simulink model "fixed_point_pi_q14"  (R2023b)
settings: Solver=FixedStepDiscrete  StartTime=0.0  StopTime=0.02  FixedStep=5.0000000000000002e-05  RelTol=1e-3
values from neighbouring files (symbols this model uses):
  feedback_step = 0.2    [build_fixed_point_pi_q14_model.m]
  kidt = Ki * Ts    (= 0.005)    [build_fixed_point_pi_q14_model.m]
  Kp = 10    [build_fixed_point_pi_q14_model.m]
  ref_step = 1.0    (= 1)    [build_fixed_point_pi_q14_model.m]
  Ts = 0.00005    (= 5e-05)    [build_fixed_point_pi_local_q_model.m]    (also in build_fixed_point_pi_q14_model.m)
  Umax = 1.8    [build_fixed_point_pi_q14_model.m]
  Umin = -1.8    [build_fixed_point_pi_q14_model.m]
settings Model: Creator=user  LastModifiedBy=user
settings OptimizationCC: DefaultParameterBehavior=Inlined  EnhancedBackFolding=on  PassReuseOutputArgsAs=Individual arguments  ZeroExternalMemoryAtStartup=off  ZeroInternalMemoryAtStartup=off  OptimizeBlockOrder=speed  DifferentSizesBufferReuse=on  OptimizationCustomize=off  EfficientTunableParamExpr=on
settings DebuggingCC: ParameterTunabilityLossMsg=error
settings HardwareCC: ProdBitPerPointer=32  ProdBitPerSizeT=32  ProdBitPerPtrDiffT=32  ProdLargestAtomicInteger=Long  ProdLargestAtomicFloat=Double  ProdWordSize=32  ProdHWDeviceType=ARM Compatible->ARM Cortex  TargetLargestAtomicInteger=Long  TargetLargestAtomicFloat=Double  TargetIntDivRoundTo=Zero  TargetEndianess=LittleEndian  TargetHWDeviceType=ARM Compatible->ARM Cortex  ProdEqTarget=off
settings SFSimCC: MATLABDynamicMemAlloc=off
settings RTWCC: Description=Embedded Coder  SystemTargetFile=ert.tlc  GenCodeOnly=on  TemplateMakefile=ert_default_tmf  GenerateReport=on
settings CodeAppCC: ForceParamTrailComments=on  IgnoreCustomStorageClasses=off  OperatorAnnotations=on  SimulinkDataObjDesc=on  SFDataObjDesc=on  InsertBlockDesc=on
settings ERTTargetCC: TargetLangStandard=C99 (ISO)  GenerateSampleERTMain=on  InlinedParameterPlacement=NonHierarchical  ERTCustomFileTemplate=example_file_process.tlc

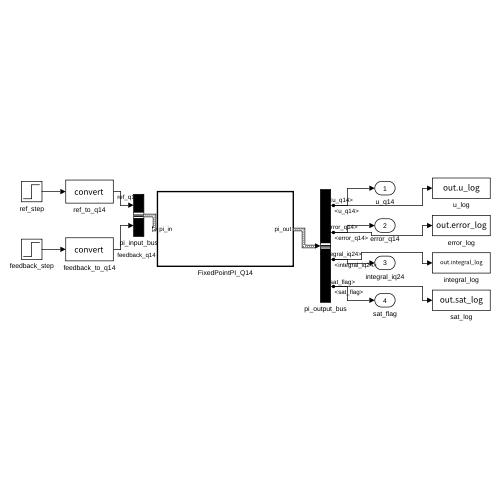
[thumbnail: Simulink's stored preview of the top-level diagram]
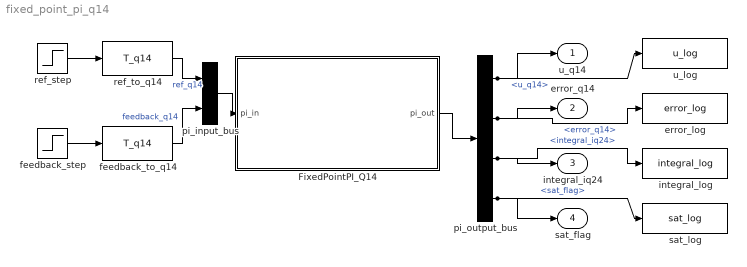
== system fixed_point_pi_q14 ==
  FixedPointPI_Q14 : Subsystem  TreatAsAtomicUnit=on
  error_log : ToWorkspace  VariableName=error_log  SaveFormat=Timeseries  SampleTime=-1
  feedback_step : Step  Time=0.006  After=feedback_step  SampleTime=Ts
  feedback_to_q14 : DataTypeConversion  OutDataTypeStr=T_q14  RndMeth=Floor
  integral_log : ToWorkspace  VariableName=integral_log  SaveFormat=Timeseries  SampleTime=-1
  pi_input_bus : BusCreator  Inputs=2  OutDataTypeStr=Bus: FixedPointPI_Q14_Input  NonVirtualBus=on
  pi_output_bus : BusSelector  OutputSignals=u_q14,error_q14,integral_iq24,sat_flag
  ref_step : Step  Time=0.001  After=ref_step  SampleTime=Ts
  ref_to_q14 : DataTypeConversion  OutDataTypeStr=T_q14  RndMeth=Floor
  sat_log : ToWorkspace  VariableName=sat_log  SaveFormat=Timeseries  SampleTime=-1
  u_log : ToWorkspace  VariableName=u_log  SaveFormat=Timeseries  SampleTime=-1
  u_q14 : Outport
  error_q14 : Outport  Port=2
  integral_iq24 : Outport  Port=3
  sat_flag : Outport  Port=4
  wires:
  ref_step/1 -> ref_to_q14/1
  feedback_step/1 -> feedback_to_q14/1
  ref_to_q14/1 -> pi_input_bus/1  "ref_q14"
  feedback_to_q14/1 -> pi_input_bus/2  "feedback_q14"
  pi_input_bus/1 -> FixedPointPI_Q14/1(pi_in)
  FixedPointPI_Q14/1(pi_out) -> pi_output_bus/1
  pi_output_bus/1 -> u_q14/1, u_log/1  "<u_q14>"
  pi_output_bus/2 -> error_q14/1, error_log/1  "<error_q14>"
  pi_output_bus/3 -> integral_iq24/1, integral_log/1  "<integral_iq24>"
  pi_output_bus/4 -> sat_flag/1, sat_log/1  "<sat_flag>"

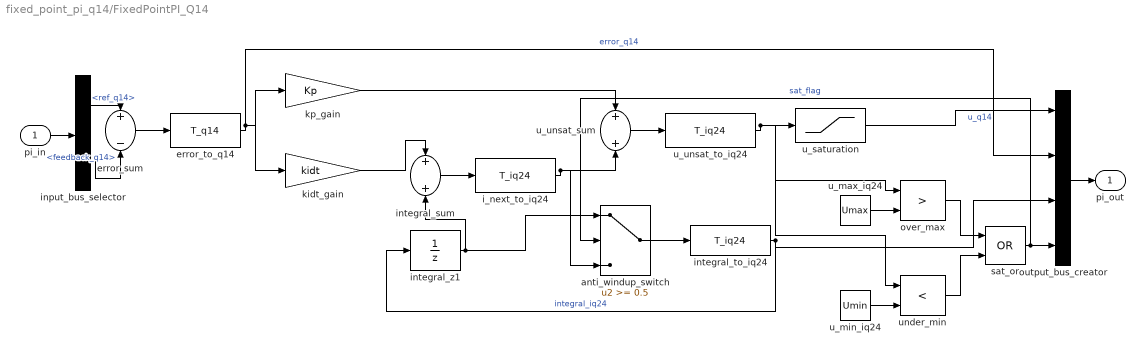
== system fixed_point_pi_q14/FixedPointPI_Q14 ==
  pi_in : Inport  OutDataTypeStr=Bus: FixedPointPI_Q14_Input
  anti_windup_switch : Switch  Threshold=0.5  SaturateOnIntegerOverflow=off  InputSameDT=off
  error_sum : Sum  Inputs=+-  OutDataTypeStr=T_q14  AccumDataTypeStr=T_iq24  SaturateOnIntegerOverflow=on
  error_to_q14 : DataTypeConversion  OutDataTypeStr=T_q14  RndMeth=Floor
  i_next_to_iq24 : DataTypeConversion  OutDataTypeStr=T_iq24  RndMeth=Floor
  input_bus_selector : BusSelector  OutputSignals=ref_q14,feedback_q14
  integral_sum : Sum  OutDataTypeStr=T_iq24  AccumDataTypeStr=T_iq24  SaturateOnIntegerOverflow=on
  integral_to_iq24 : DataTypeConversion  OutDataTypeStr=T_iq24  RndMeth=Floor
  integral_z1 : UnitDelay  SampleTime=Ts  HasFrameUpgradeWarning=on
  kidt_gain : Gain  Gain=kidt  ParamDataTypeStr=T_gain  OutDataTypeStr=T_iq24  SaturateOnIntegerOverflow=on
  kp_gain : Gain  Gain=Kp  ParamDataTypeStr=T_gain  OutDataTypeStr=T_iq24  SaturateOnIntegerOverflow=on
  output_bus_creator : BusCreator  Inputs=4  OutDataTypeStr=Bus: FixedPointPI_Q14_Output  NonVirtualBus=on
  over_max : RelationalOperator  Operator=>  OutDataTypeStr=boolean  RndMeth=Simplest  InputSameDT=off
  sat_or : Logic  Operator=OR  AllPortsSameDT=off  OutDataTypeStr=boolean
  u_max_iq24 : Constant  Value=Umax  OutDataTypeStr=T_iq24
  u_min_iq24 : Constant  Value=Umin  OutDataTypeStr=T_iq24
  u_saturation : Saturate  UpperLimit=Umax  LowerLimit=Umin  OutDataTypeStr=T_q14
  u_unsat_sum : Sum  OutDataTypeStr=T_iq24  AccumDataTypeStr=T_iq24  SaturateOnIntegerOverflow=on
  u_unsat_to_iq24 : DataTypeConversion  OutDataTypeStr=T_iq24  RndMeth=Floor
  under_min : RelationalOperator  Operator=<  OutDataTypeStr=boolean  RndMeth=Simplest  InputSameDT=off
  pi_out : Outport  OutDataTypeStr=Bus: FixedPointPI_Q14_Output
  wires:
  pi_in/1 -> input_bus_selector/1
  input_bus_selector/1 -> error_sum/1  "<ref_q14>"
  input_bus_selector/2 -> error_sum/2  "<feedback_q14>"
  error_sum/1 -> error_to_q14/1
  error_to_q14/1 -> kp_gain/1, kidt_gain/1, output_bus_creator/2  "error_q14"
  kidt_gain/1 -> integral_sum/1
  integral_z1/1 -> integral_sum/2, anti_windup_switch/1
  integral_sum/1 -> i_next_to_iq24/1
  kp_gain/1 -> u_unsat_sum/1
  i_next_to_iq24/1 -> u_unsat_sum/2, anti_windup_switch/3
  u_unsat_sum/1 -> u_unsat_to_iq24/1
  u_unsat_to_iq24/1 -> u_saturation/1, over_max/1, under_min/1
  u_max_iq24/1 -> over_max/2
  u_min_iq24/1 -> under_min/2
  over_max/1 -> sat_or/1
  under_min/1 -> sat_or/2
  sat_or/1 -> anti_windup_switch/2, output_bus_creator/4  "sat_flag"
  anti_windup_switch/1 -> integral_to_iq24/1
  integral_to_iq24/1 -> integral_z1/1, output_bus_creator/3  "integral_iq24"
  u_saturation/1 -> output_bus_creator/1  "u_q14"
  output_bus_creator/1 -> pi_out/1
